simulink model "robotManipulatorModel"  (R2024a)
settings: Solver=FixedStepAuto  StartTime=0.0  StopTime=10  FixedStep=1e-3  RelTol=1e-3
undefined symbols (not defined in the file): a1, a2, b1, b2, C, c1, c2, D, d1, d2, delta, eta, J1, J2, Jd1, Jd2, K, L1, L2, Ld1, Ld2, M1, M2, Md1, Md2, Phi, x0
settings Model: Creator=The MathWorks, Inc.  LastModifiedBy=The MathWorks, Inc.
settings RTWCC: GPUComputeCapability=3.5

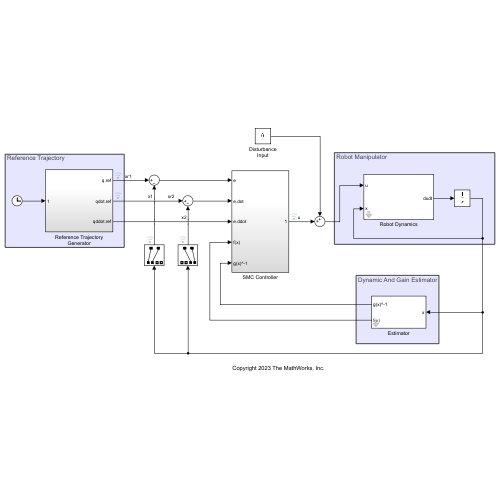
[thumbnail: Simulink's stored preview of the top-level diagram]
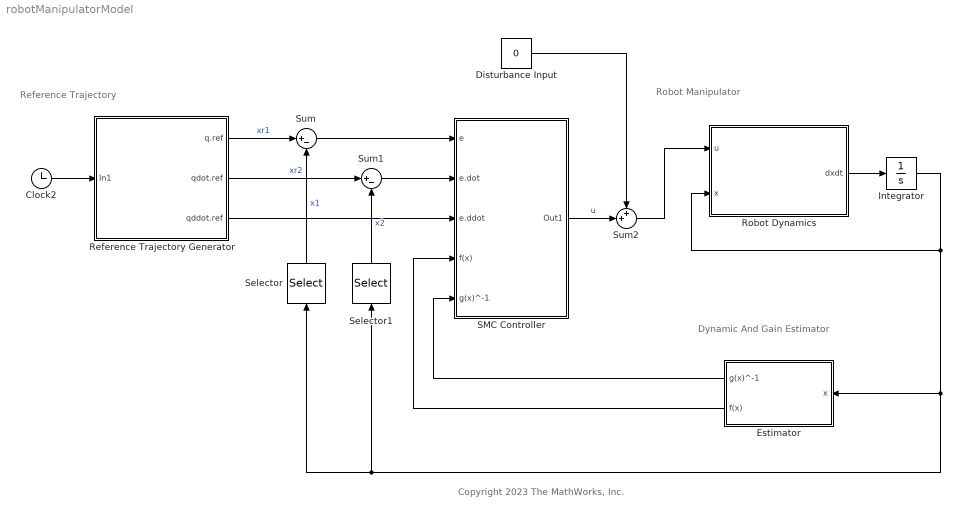
== system robotManipulatorModel ==
  note: Dynamic And Gain Estimator
  note: Reference Trajectory
  note: Robot Manipulator
  note: Copyright 2023 The MathWorks, Inc.
  Clock2 : Clock
  Disturbance Input : Constant  Value=0
  Estimator : Subsystem  mask{m1=Md1, m2=Md2, r1=Ld1, r2=Ld2, J1=Jd1, J2=Jd2, g=9.81}
      mask prompts: m1 "Mass 1"; m2 "Mass 2"; r1 "Link length 1"; r2 "Link length 2"; J1 "Inertia 1"; J2 "Inertia 2"; g "Gravity constant"
      mask DialogControl DescTextVar Prompt:
      | This block calculates the mass matrix, M, Coriolis and centrifugal matrix, C, and gravity vector, G for a Two-joint robotic arm, based on the current joint angles, velocities, and a set of user-defined physical parameters.
      | 
      |  Modify the physical parameters to analyze the robustness of the Sliding Mode Control (SMC) controller across different robotic arm configurations.
  Integrator : Integrator  InitialCondition=x0
  Reference Trajectory Generator : Subsystem
  Robot Dynamics : Subsystem  mask{m1=M1, m2=M2, r1=L1, r2=L2, J1=J1, J2=J2, g=9.81}
      mask prompts: m1 "Mass 1"; m2 "Mass 2"; r1 "Link length 1"; r2 "Link length 2"; J1 "Inertia 1"; J2 "Inertia 2"; g "Gravity constant"
      mask DialogControl DescTextVar Prompt: This block computes the state derivatives of a Two-joint robotic arm model based on input torques and user-defined physical parameters.
  SMC Controller : Subsystem
  Selector : Selector  InputPortWidth=4  IndexOptions=Index vector (dialog)  Indices=[1 2]  OutputSizes=1
  Selector1 : Selector  InputPortWidth=4  IndexOptions=Index vector (dialog)  Indices=[3 4]  OutputSizes=1
  Sum : Sum  Inputs=|+-
  Sum1 : Sum  Inputs=|+-
  Sum2 : Sum  Inputs=++|
  wires:
  Sum/1 -> SMC Controller/1(e)
  Sum1/1 -> SMC Controller/2(e.dot)
  Selector1/1 -> Sum1/2  "x2"
  Selector/1 -> Sum/2  "x1"
  SMC Controller/1(Out1) -> Sum2/2  "u"
  Disturbance Input/1 -> Sum2/1
  Sum2/1 -> Robot Dynamics/1(u)
  Robot Dynamics/1(dxdt) -> Integrator/1
  Reference Trajectory Generator/3(qddot.ref) -> SMC Controller/3(e.ddot)
  Reference Trajectory Generator/1(q.ref) -> Sum/1  "xr1"
  Reference Trajectory Generator/2(qdot.ref) -> Sum1/1  "xr2"
  Clock2/1 -> Reference Trajectory Generator/1(In1)
  Estimator/1(g(x)^-1) -> SMC Controller/5(g(x)^-1)
  Estimator/2(f(x)) -> SMC Controller/4(f(x))
  Integrator/1 -> Selector1/1, Selector/1, Estimator/1(x), Robot Dynamics/2(x)

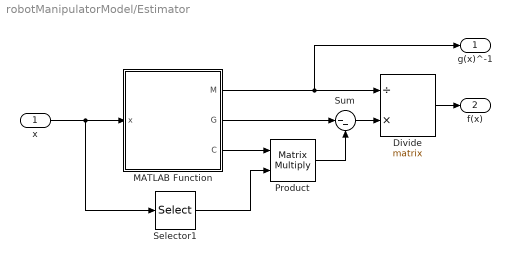
== system robotManipulatorModel/Estimator ==
  x : Inport
  Divide : Product  Inputs=/*  Multiplication=Matrix(*)
  MATLAB Function : MATLAB Function  TreatAsAtomicUnit=on
  Product : Product  Multiplication=Matrix(*)
  Selector1 : Selector  InputPortWidth=4  IndexOptions=Index vector (dialog)  Indices=[3 4]  OutputSizes=1
  Sum : Sum  Inputs=|--
  g(x)^-1 : Outport
  f(x) : Outport  Port=2
  wires:
  x/1 -> MATLAB Function/1(x), Selector1/1
  MATLAB Function/1(M) -> g(x)^-1/1, Divide/1
  MATLAB Function/3(C) -> Product/1
  Selector1/1 -> Product/2
  Divide/1 -> f(x)/1
  MATLAB Function/2(G) -> Sum/1
  Product/1 -> Sum/2
  Sum/1 -> Divide/2

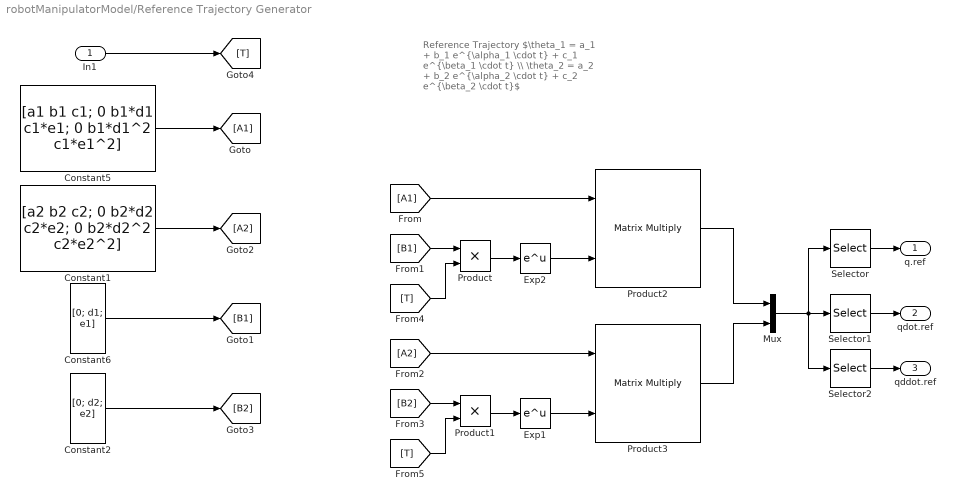
== system robotManipulatorModel/Reference Trajectory Generator ==
  note: Reference Trajectory
      |
      | $\theta_1 = a_1 + b_1 e^{\alpha_1 \cdot t} + c_1 e^{\beta_1 \cdot t} \\ \theta_2 = a_2 + b_2 e^{\alpha_2 \cdot t} + c_2 e^{\beta_2 \cdot t}$
  In1 : Inport
  Constant1 : Constant  Value=[a2 b2 c2; 0 b2*d2 c2*e2; 0 b2*d2^2 c2*e2^2]  VectorParams1D=off
  Constant2 : Constant  Value=[0; d2; e2]  VectorParams1D=off
  Constant5 : Constant  Value=[a1 b1 c1; 0 b1*d1 c1*e1; 0 b1*d1^2 c1*e1^2]  VectorParams1D=off
  Constant6 : Constant  Value=[0; d1; e1]  VectorParams1D=off
  Exp1 : Math
  Exp2 : Math
  Mux : Mux  Inputs=2
  Product : Product
  Product1 : Product
  Product2 : Product  Multiplication=Matrix(*)
  Product3 : Product  Multiplication=Matrix(*)
  Selector : Selector  InputPortWidth=6  IndexOptions=Index vector (dialog)  Indices=[1 4]  OutputSizes=1
  Selector1 : Selector  InputPortWidth=6  IndexOptions=Index vector (dialog)  Indices=[2 5]  OutputSizes=1
  Selector2 : Selector  InputPortWidth=6  IndexOptions=Index vector (dialog)  Indices=[3 6]  OutputSizes=1
  q.ref : Outport
  qdot.ref : Outport  Port=2
  qddot.ref : Outport  Port=3
  wires:
  Exp2/1 -> Product2/2
  Product/1 -> Exp2/1
  Constant5/1 -> [A1]
  [A1] -> Product2/1
  Constant6/1 -> [B1]
  [B1] -> Product/1
  Constant2/1 -> [B2]
  Constant1/1 -> [A2]
  In1/1 -> [T]
  [T] -> Product/2
  [B2] -> Product1/1
  Product1/1 -> Exp1/1
  [A2] -> Product3/1
  Exp1/1 -> Product3/2
  [T] -> Product1/2
  Mux/1 -> Selector2/1, Selector1/1, Selector/1
  Product2/1 -> Mux/1
  Product3/1 -> Mux/2
  Selector/1 -> q.ref/1
  Selector1/1 -> qdot.ref/1
  Selector2/1 -> qddot.ref/1

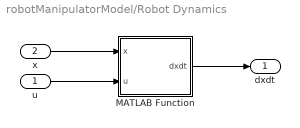
== system robotManipulatorModel/Robot Dynamics ==
  u : Inport
  x : Inport  Port=2
  MATLAB Function : MATLAB Function  TreatAsAtomicUnit=on
  dxdt : Outport
  wires:
  MATLAB Function/1(dxdt) -> dxdt/1
  x/1 -> MATLAB Function/1(x)
  u/1 -> MATLAB Function/2(u)

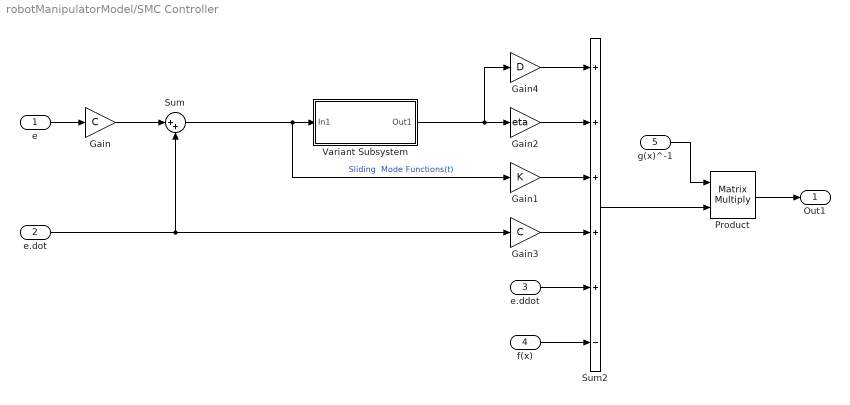
== system robotManipulatorModel/SMC Controller ==
  e : Inport
  e.dot : Inport  Port=2
  e.ddot : Inport  Port=3
  f(x) : Inport  Port=4
  g(x)^-1 : Inport  Port=5
  Gain : Gain  Gain=C
  Gain1 : Gain  Gain=K
  Gain2 : Gain  Gain=eta
  Gain3 : Gain  Gain=C
  Gain4 : Gain  Gain=D
  Product : Product  Multiplication=Matrix(*)
  Sum : Sum  Inputs=|++
  Sum2 : Sum  Inputs=+++++-
  Variant Subsystem : Subsystem  Variant=on  VariantControlMode=label  LabelModeActiveChoice=saturation  mask{VChoice=sign}
      mask prompts: VChoice "Select Switching Function"
      mask TypeOptions VChoice: sign | saturation | relay
      mask DialogControl DescTextVar Prompt:
      | This block calculates the mass matrix, M, Coriolis and centrifugal matrix, C, and gravity vector, G for a Two-joint robotic arm, based on the current joint angles, velocities, and a set of user-defined physical parameters.
      | 
      |  Modify the physical parameters to analyze the robustness of the Sliding Mode Control (SMC) controller across different robotic arm configurations.
  Out1 : Outport
  wires:
  e/1 -> Gain/1
  Gain/1 -> Sum/1
  e.dot/1 -> Sum/2, Gain3/1
  Sum/1 -> Variant Subsystem/1(In1), Gain1/1  "Sliding  Mode Functions(t)"
  Product/1 -> Out1/1
  Sum2/1 -> Product/2
  g(x)^-1/1 -> Product/1
  f(x)/1 -> Sum2/6
  e.ddot/1 -> Sum2/5
  Gain3/1 -> Sum2/4
  Gain2/1 -> Sum2/2
  Gain1/1 -> Sum2/3
  Variant Subsystem/1(Out1) -> Gain4/1, Gain2/1
  Gain4/1 -> Sum2/1

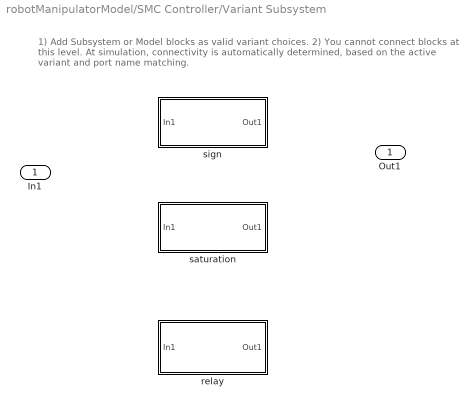
== system robotManipulatorModel/SMC Controller/Variant Subsystem ==
  note: 1) Add Subsystem or Model blocks as valid variant choices.
      | 2) You cannot connect blocks at this level. At simulation, connectivity is automatically
      | determined, based on the active variant and port name matching.
  In1 : Inport
  relay : Subsystem  VariantControl=relay
  saturation : Subsystem  VariantControl=saturation
  sign : Subsystem  VariantControl=sign
  Out1 : Outport

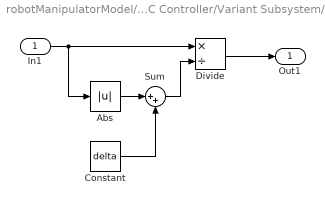
== system robotManipulatorModel/SMC Controller/Variant Subsystem/relay ==
  In1 : Inport
  Abs : Abs  SaturateOnIntegerOverflow=off
  Constant : Constant  Value=delta
  Divide : Product  Inputs=*/
  Sum : Sum  Inputs=|++
  Out1 : Outport
  wires:
  Divide/1 -> Out1/1
  In1/1 -> Divide/1, Abs/1
  Sum/1 -> Divide/2
  Abs/1 -> Sum/1
  Constant/1 -> Sum/2

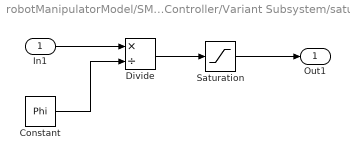
== system robotManipulatorModel/SMC Controller/Variant Subsystem/saturation ==
  In1 : Inport
  Constant : Constant  Value=Phi  VectorParams1D=off
  Divide : Product  Inputs=*/
  Saturation : Saturate
  Out1 : Outport
  wires:
  Saturation/1 -> Out1/1
  Divide/1 -> Saturation/1
  In1/1 -> Divide/1
  Constant/1 -> Divide/2

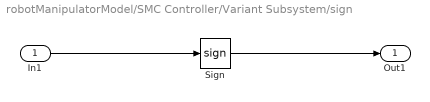
== system robotManipulatorModel/SMC Controller/Variant Subsystem/sign ==
  In1 : Inport
  Sign : Signum  ZeroCross=off
  Out1 : Outport
  wires:
  In1/1 -> Sign/1
  Sign/1 -> Out1/1

== matlab function robotManipulatorModel/Estimator/MATLAB Function ==
  data: M output; G output; C output; x input; m1 parameter; m2 parameter; r1 parameter; r2 parameter; J1 parameter; J2 parameter; g parameter
function [M, G, C] = fcn(x, m1, m2, r1, r2, J1, J2, g)

param.m1 = m1; % Mass 1
param.m2 = m2; % Mass 2
param.r1 = r1; % Link length 1
param.r2 = r2; % Link length 2
param.J1 = J1; % Inertia 1
param.J2 = J2; % Inertia 2
param.g  = g;  % Gravity constant

M = zeros(2,2,'like', x);
C = zeros(2,2,'like', x);
G = zeros(2,1,'like', x);

[~, M, C, G] = robotStateFcn(x, zeros(2,1), param);

== matlab function robotManipulatorModel/Robot Dynamics/MATLAB Function ==
  data: x input; u input; m1 parameter; m2 parameter; r1 parameter; r2 parameter; J1 parameter; J2 parameter; dxdt output; g parameter
function dxdt = fcn(x, u, m1, m2, r1, r2, J1, J2, g)

param.m1 = m1; % Mass 1
param.m2 = m2; % Mass 2
param.r1 = r1; % Link length 1
param.r2 = r2; % Link length 2
param.J1 = J1; % Inertia 1
param.J2 = J2; % Inertia 2
param.g  = g;  % Gravity constant

dxdt = zeros(4,1,'like', x);
dxdt = robotStateFcn(x, u, param);
